simulink model "InProgressPIDController"  (R2023b)
settings: Solver=VariableStepAuto  StartTime=0.0  StopTime=10.0  RelTol=1e-3
undefined symbols (not defined in the file): Kd, Ki, Kp, m, x_d
settings Model: Creator=billy  LastModifiedBy=billy

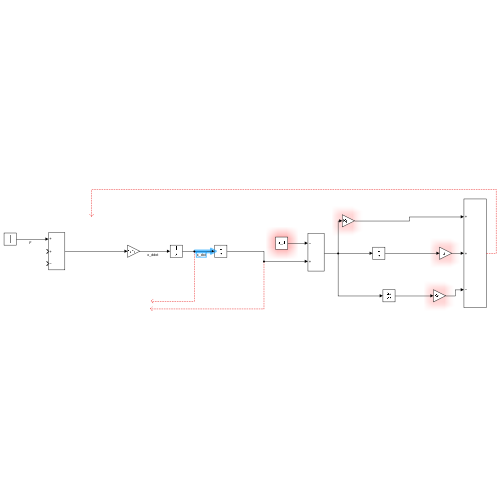
[thumbnail: Simulink's stored preview of the top-level diagram]
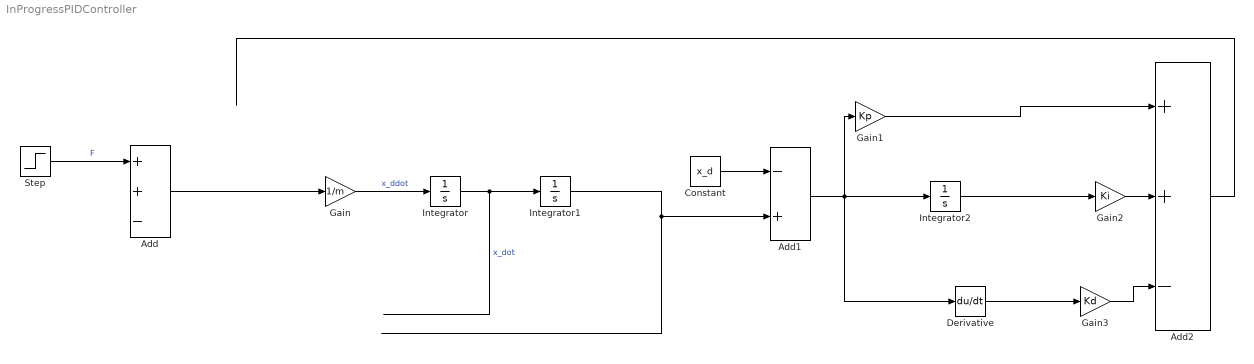
== system InProgressPIDController ==
  Add : Sum  Inputs=++-
  Add1 : Sum  Inputs=-+
  Add2 : Sum  Inputs=++-
  Constant : Constant  Value=x_d
  Derivative : Derivative
  Gain : Gain  Gain=1/m
  Gain1 : Gain  Gain=Kp
  Gain2 : Gain  Gain=Ki
  Gain3 : Gain  Gain=Kd
  Integrator : Integrator
  Integrator1 : Integrator
  Integrator2 : Integrator
  Step : Step  SampleTime=0
  wires:
  Step/1 -> Add/1  "F"
  Add/1 -> Gain/1
  Gain/1 -> Integrator/1  "x_ddot"
  Integrator/1 -> Integrator1/1  "x_dot"
  Integrator1/1 -> Add1/2
  Constant/1 -> Add1/1
  Add1/1 -> Derivative/1, Integrator2/1, Gain1/1
  Integrator2/1 -> Gain2/1
  Gain1/1 -> Add2/1
  Gain2/1 -> Add2/2
  Derivative/1 -> Gain3/1
  Gain3/1 -> Add2/3
  Add2/1 -> ?
